simulink model "Dynamic"  (R2023b)
settings: Solver=VariableStepAuto  StartTime=0.0  StopTime=10  RelTol=1e-3
values from neighbouring files (symbols this model uses):
  D = x(19)    [BSM.m]    (also in Correct_new_data.m; GenerateSimplifiedMechanism.m; MechanicalMechanics_Dynamic_adaptive_BSM.m; MechanicalMechanics_Kinematics.m)
  ddQ1 = x(7)    [Adams_HW1.m]    (also in BSM.m; Correct_new_data.m; MechanicalMechanics_Dynamic.m; MechanicalMechanics_Dynamic_adaptive_BSM.m)
  L1 = x(1)    [Adams_HW1.m]    (also in Adams_HW_DrawGIF.m = current_x(1); Adams_HW_DrawGIF_Y.m = current_x(1); BSM.m; Correct_new_data.m)
  L2 = x(2)    [Adams_HW1.m]    (also in Adams_HW_DrawGIF.m = current_x(2); Adams_HW_DrawGIF_Y.m = current_x(2); BSM.m; Correct_new_data.m)
  L3 = x(3)    [Adams_HW1.m]    (also in Adams_HW_DrawGIF.m = current_x(3); Adams_HW_DrawGIF_Y.m = current_x(3); BSM.m; Correct_new_data.m)
  L4 = x(4)    [Adams_HW1.m]    (also in Adams_HW_DrawGIF.m = current_x(4); Adams_HW_DrawGIF_Y.m = current_x(4); BSM.m; Correct_new_data.m)
  Q1 = x(5)    [Adams_HW1.m]    (also in Adams_HW_DrawGIF.m = current_x(5); Adams_HW_DrawGIF_Y.m = current_x(5); BSM.m; Correct_new_data.m)
  Q2 = Inition(1)    [Adams_HW1.m]    (also in BSM.m = x(8); Correct_new_data.m = x(8); GenerateSimplifiedMechanism.m = x(8); MechanicalMechanics_Dynamic.m = x(8))
  Q3 = x(11)    [Adams_HW1.m]    (also in Adams_HW_DrawGIF.m = current_x(11); Adams_HW_DrawGIF_Y.m = current_x(7); BSM.m; Correct_new_data.m)
  s = x(14)    [BSM.m]    (also in Correct_new_data.m; GenerateSimplifiedMechanism.m; MechanicalMechanics_Dynamic.m; MechanicalMechanics_Dynamic_adaptive_BSM.m)
settings Model: Creator=Akko  LastModifiedBy=Akko

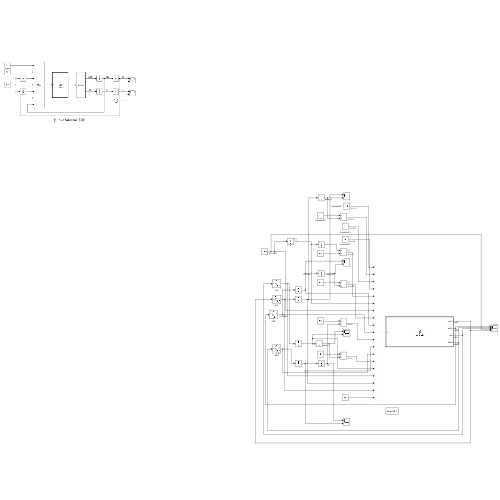
[thumbnail: Simulink's stored preview of the top-level diagram]
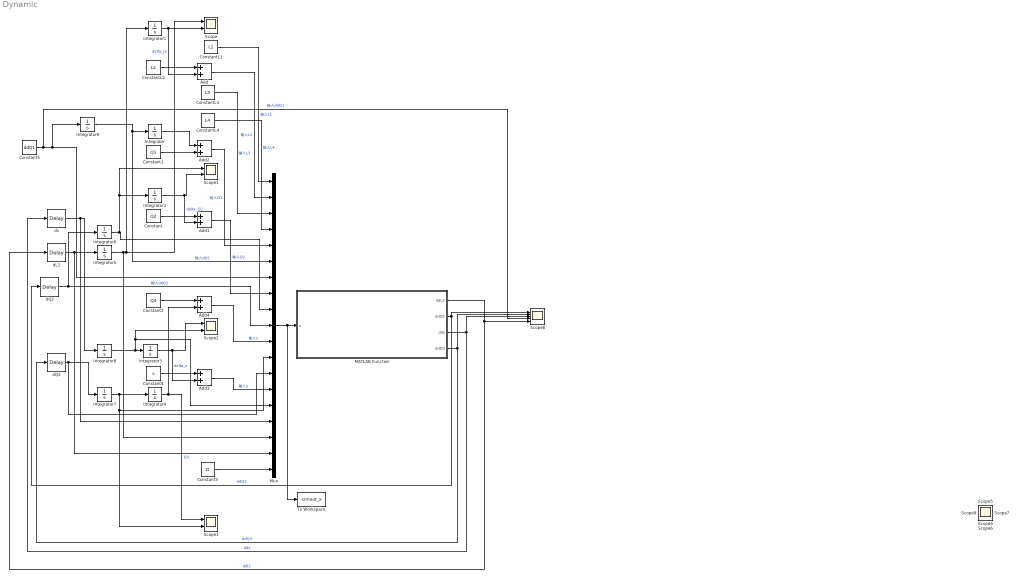
== system Dynamic ==
  Add{,1..4} (5 alike) : Sum
  Constant : Constant  Value=Q2
  Constant1 : Constant  Value=Q1
  Constant2 : Constant  Value=Q3
  Constant3 : Constant  Value=D
  Constant5 : Constant  Value=ddQ1
  Constant8 : Constant  Value=s
  ConstantL1 : Constant  Value=L1
  ConstantL2 : Constant  Value=L2
  ConstantL3 : Constant  Value=L3
  ConstantL4 : Constant  Value=L4
  Integrator{,1..9} (10 alike) : Integrator
  MATLAB Function : MATLAB Function  TreatAsAtomicUnit=on
  Mux : Mux  Inputs=19
  Scope{,1..3} (4 alike) : Scope  NumInputPorts=2
  Scope8 : Scope  NumInputPorts=5
  To Workspace : ToWorkspace  VariableName=simout_x  SampleTime=-1
  dL2 : TransportDelay  DelayTime=1e-4
  dQ2 : TransportDelay  DelayTime=1e-4
  dQ3 : TransportDelay  DelayTime=1e-4
  ds : TransportDelay  DelayTime=1e-4
  Scope{4..7,9} (5 alike) : Scope
  wires:
  ds/1 -> Mux/16, Integrator8/1
  dL2/1 -> Mux/18, Integrator5/1
  Integrator6/1 -> Scope1/1, Integrator2/1, Mux/9
  Integrator8/1 -> Scope2/2, Mux/15, Integrator3/1
  Integrator7/1 -> Mux/12, Scope3/2, Integrator4/1
  Integrator5/1 -> Scope/1, Integrator1/1, Mux/17
  dQ2/1 -> Mux/10, Integrator6/1  "输入ddQ2"
  Add2/1 -> Mux/5  "输入Q1"
  Integrator9/1 -> Mux/6, Integrator/1  "输入dQ1"
  dQ3/1 -> Mux/13, Integrator7/1
  Add3/1 -> Mux/14  "输入s"
  Integrator1/1 -> Scope/2, Add/2  "delta_l2"
  Constant/1 -> Add1/1
  ConstantL2/1 -> Add/1
  MATLAB Function/3(dds) -> ds/1, Scope8/3  "dds"
  MATLAB Function/2(ddQ2) -> dQ2/1, Scope8/1  "ddQ2"
  ConstantL4/1 -> Mux/4  "输入L4"
  Integrator/1 -> Add2/1
  Constant1/1 -> Add2/2
  Integrator2/1 -> Add1/2, Scope1/2  "delta_Q2"
  Add4/1 -> Mux/11  "输入s"
  Constant8/1 -> Add3/1
  Constant2/1 -> Add4/1
  Constant5/1 -> Scope8/4, Integrator9/1, Mux/7  "输入ddQ1"
  Integrator4/1 -> Scope3/1, Add4/2  "Q3"
  Integrator3/1 -> Add3/2, Scope2/1  "delta_s"
  ConstantL3/1 -> Mux/3  "输入L3"
  ConstantL1/1 -> Mux/1  "输入L1"
  MATLAB Function/1(ddL2) -> dL2/1, Scope8/5  "ddl2"
  Add/1 -> Mux/2  "输入L2"
  Add1/1 -> Mux/8  "输入Q2"
  Constant3/1 -> Mux/19
  Mux/1 -> MATLAB Function/1(u), To Workspace/1
  MATLAB Function/4(ddQ3) -> dQ3/1, Scope8/2  "ddQ3"

== matlab function Dynamic/MATLAB Function ==
  data: u input; ddL2 output; ddQ2 output; dds output; ddQ3 output
function [ddL2,ddQ2,dds,ddQ3]=Dynamic(u)
coder.extrinsic('MechanicalMechanics_Dynamic');
ddL2 = 0; ddQ2 = 0; dds = 0; ddQ3 = 0;
[ddL2,ddQ2,dds,ddQ3] = MechanicalMechanics_Kinematics(u);
end
